simulink model "MicroGrid"  (R2021a)
settings: Solver=VariableStepAuto  StartTime=0  StopTime=24*3600  RelTol=1e-3
values from neighbouring files (symbols this model uses):
  A = A_prWindturbine * number_of_windturbines    (= 1530247.6)    [load_global_variables.m]
  Area_panels = 5*number_households    (= 1000000)    [load_global_variables.m]
  Battery_Capacity = 100e3    (= 100000)    [load_global_variables.m]
  controller_delay = 5    [load_global_variables.m]
  Efficiency_solar = 0.1    [load_global_variables.m]
  Efficiency_wind = 0.4    [load_global_variables.m]
  fuel_cell_power_rating = 50e6*4    (= 200000000)    [load_global_variables.m]
  H2_safety_buffer = 50e6    (= 50000000)    [load_global_variables.m]
  H2_selfsupply = 100e6    (= 100000000)    [load_global_variables.m]
  Max_H2_P_Input = 260000000    [load_global_variables.m]
  maxSOC = 100    [load_global_variables.m]
  Min_H2_P_Input = 1400    [load_global_variables.m]
  minSOC = 60    [load_global_variables.m]
  number_cars = number_households/3    (= 66666.6666667)    [load_global_variables.m]
  number_households = 200000    [load_global_variables.m]
  number_of_windturbines = 35    [load_global_variables.m]
  P_charge_max = 250e3    (= 250000)    [load_global_variables.m]
  P_rating_bat_single = 14e3    (= 14000)    [load_global_variables.m]
  Rho = 1.204    [load_global_variables.m]
  scenario = 5    [load_global_variables.m]
  SOC_safety_buffer = 80    [load_global_variables.m]
  SOC_selfsupply = 90    [load_global_variables.m]
  SOC_Start = 60    [load_global_variables.m]
  Start_Tank_Fill_L = 50e6    (= 50000000)    [load_global_variables.m]
  SunWinter = [0 0 0 0 0 0 0 33.54 130.49 211.47 234.96 271.04 ... (24 elements, 1x24)]    [SunWinter.mat]
undefined symbols (not defined in the file or in its folder): EV_dist, price, SunFall, SunSpring, SunSummer, Vind15nov, Vind23sep, wind
settings Model: Creator=cm  LastModifiedBy=cm

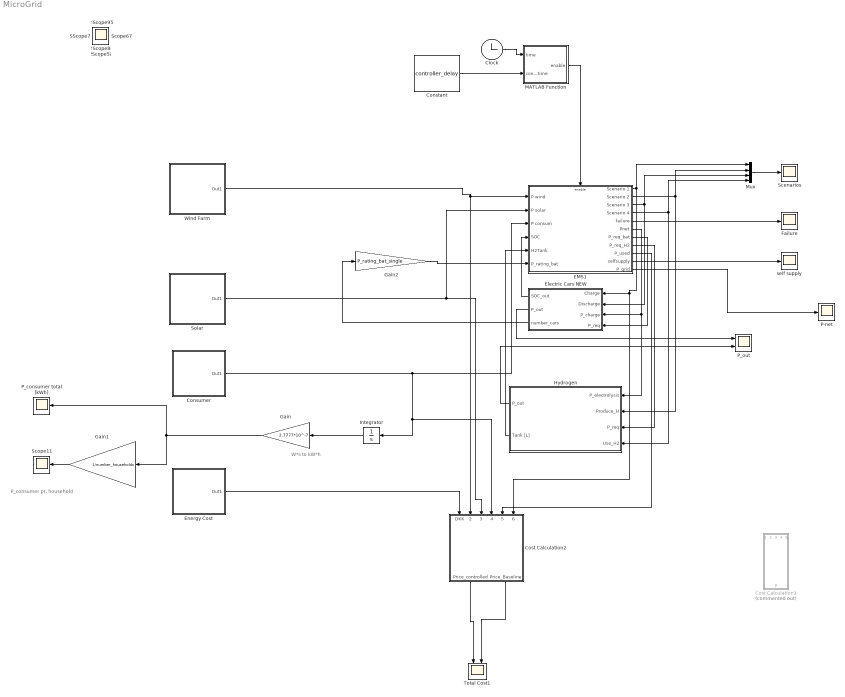
== system MicroGrid ==
  note: W*s to kW*h
  note: P_consumer pr. household
  Clock : Clock
  Constant : Constant  Value=controller_delay
  Consumer : Subsystem
      mask Display: image('C:\Users\cm\OneDrive - Danmarks Tekniske Universitet\Model-Based Systems Eng\05 Models\MBSE-MicroGrid\OurModel\Icons\House.png'); % Use "Edit Image" on toolstrip to change.
  Cost Calculation1 : Subsystem  Commented=on
  Cost Calculation2 : Subsystem
  EMS1 : Subsystem
  Electric Cars NEW : Subsystem
  Energy Cost : Subsystem
      mask Display: image('C:\Users\cm\OneDrive - Danmarks Tekniske Universitet\Model-Based Systems Eng\05 Models\MBSE-MicroGrid\OurModel\Icons\el_cost.png'); % Use "Edit Image" on toolstrip to change.
  Failure : Scope
  Gain : Gain  Gain=2.7777*10^-7
  Gain1 : Gain  Gain=1/number_households
  Gain2 : Gain  Gain=P_rating_bat_single
  Hydrogen : Subsystem
  Integrator : Integrator
  MATLAB Function : MATLAB Function  TreatAsAtomicUnit=on
  Mux : Mux
  P-net : Scope
  P_consumer total [kWh] : Scope
  P_out : Scope  NumInputPorts=2
  Scenarios : Scope
  Scope{,1..17} (18 alike) : Scope
  Solar : Subsystem
      mask Display: image('C:\Users\cm\OneDrive - Danmarks Tekniske Universitet\Model-Based Systems Eng\05 Models\MBSE-MicroGrid\OurModel\Icons\solar.png'); % Use "Edit Image" on toolstrip to change.
  Total Cost1 : Scope  NumInputPorts=2
  Wind Farm : Subsystem
      mask Display: image('C:\Users\cm\OneDrive - Danmarks Tekniske Universitet\Model-Based Systems Eng\05 Models\MBSE-MicroGrid\OurModel\Icons\wind.png'); % Use "Edit Image" on toolstrip to change.
  self supply : Scope
  wires:
  Electric Cars NEW/2(P_out) -> P_out/1
  Solar/1(Out1) -> Cost Calculation2/3(P solar), EMS1/2(P solar)
  EMS1/6(Pnet) -> Hydrogen/1(P_electrolysis), Electric Cars NEW/3(P_charge)
  EMS1/3(Scenario 3) -> Mux/3, Electric Cars NEW/2(Discharge)
  Hydrogen/2(Tank [L]) -> EMS1/5(H2Tank)
  Hydrogen/1(P_out) -> P_out/2
  Wind Farm/1(Out1) -> Cost Calculation2/2(P wind), EMS1/1(P wind)
  Electric Cars NEW/1(SOC_out) -> EMS1/4(SOC)
  Gain1/1 -> Scope11/1
  Gain/1 -> Gain1/1, P_consumer total [kWh]/1
  Energy Cost/1(Out1) -> Cost Calculation2/1(DKK)
  Integrator/1 -> Gain/1
  Cost Calculation2/1(Price_controlled) -> Total Cost1/1
  Consumer/1(Out1) -> EMS1/3(P consum), Cost Calculation2/4(P_consumer), Integrator/1
  Gain2/1 -> EMS1/6(P_rating_bat)
  Electric Cars NEW/3(number_cars) -> Gain2/1
  MATLAB Function/1(enable) -> EMS1/Enable
  Constant/1 -> MATLAB Function/2(controller_time)
  Clock/1 -> MATLAB Function/1(time)
  EMS1/1(Scenario 1) -> Mux/1, Cost Calculation2/6(P_cars), Electric Cars NEW/1(Charge)
  EMS1/2(Scenario 2) -> Mux/2, Hydrogen/2(Produce_H)
  EMS1/4(Scenario 4) -> Mux/4, Hydrogen/4(Use_H2)
  EMS1/5(failure) -> Failure/1
  EMS1/7(P_req_bat) -> Electric Cars NEW/4(P_req)
  EMS1/8(P_req_H2) -> Hydrogen/3(P_req)
  EMS1/10(selfsupply) -> self supply/1
  Cost Calculation2/2(Price_Baseline) -> Total Cost1/2
  EMS1/9(P_used) -> Cost Calculation2/5(P_used)
  EMS1/11(P_grid) -> P-net/1
  Mux/1 -> Scenarios/1

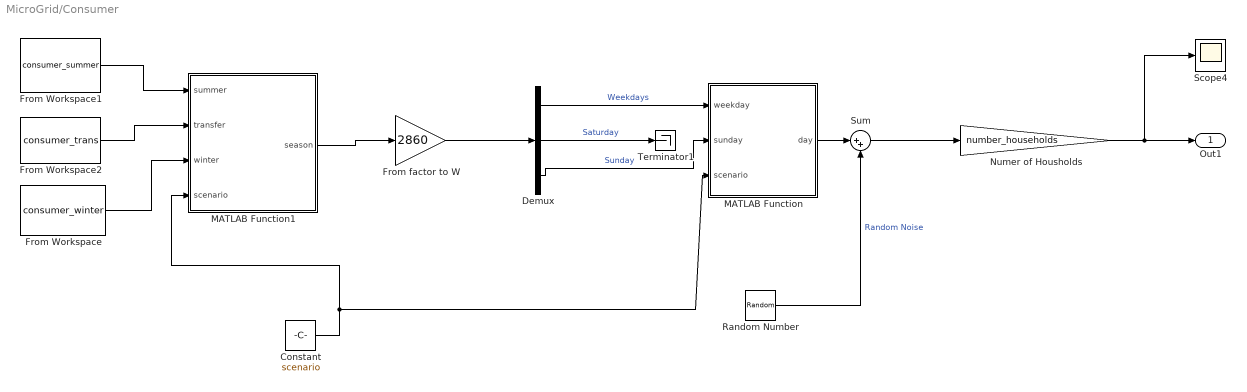
== system MicroGrid/Consumer ==
  Constant : Constant  Value=scenario
  Demux : Demux  Outputs=3
  From Workspace : FromWorkspace  VariableName=consumer_winter  SampleTime=24*60*60/96  Interpolate=off  ZeroCross=off  OutputAfterFinalValue=Cyclic repetition
  From Workspace1 : FromWorkspace  VariableName=consumer_summer  SampleTime=24*60*60/96  Interpolate=off  ZeroCross=off  OutputAfterFinalValue=Cyclic repetition
  From Workspace2 : FromWorkspace  VariableName=consumer_trans  SampleTime=24*60*60/96  Interpolate=off  ZeroCross=off  OutputAfterFinalValue=Cyclic repetition
  From factor to W : Gain  Gain=2860
  MATLAB Function : MATLAB Function  TreatAsAtomicUnit=on
  MATLAB Function1 : MATLAB Function  TreatAsAtomicUnit=on
  Numer of Housholds : Gain  Gain=number_households
  Random Number : RandomNumber  Variance=0.0001  SampleTime=1*60*60
  Scope4 : Scope
  Sum : Sum  Inputs=|++
  Terminator1 : Terminator
  Out1 : Outport
  wires:
  Demux/2 -> Terminator1/1  "Saturday"
  Random Number/1 -> Sum/2  "Random Noise"
  Demux/3 -> MATLAB Function/2(sunday)  "Sunday"
  Sum/1 -> Numer of Housholds/1
  Numer of Housholds/1 -> Out1/1, Scope4/1
  From factor to W/1 -> Demux/1
  From Workspace1/1 -> MATLAB Function1/1(summer)
  From Workspace2/1 -> MATLAB Function1/2(transfer)
  From Workspace/1 -> MATLAB Function1/3(winter)
  MATLAB Function1/1(season) -> From factor to W/1
  MATLAB Function/1(day) -> Sum/1
  Demux/1 -> MATLAB Function/1(weekday)  "Weekdays"
  Constant/1 -> MATLAB Function/3(scenario), MATLAB Function1/4(scenario)

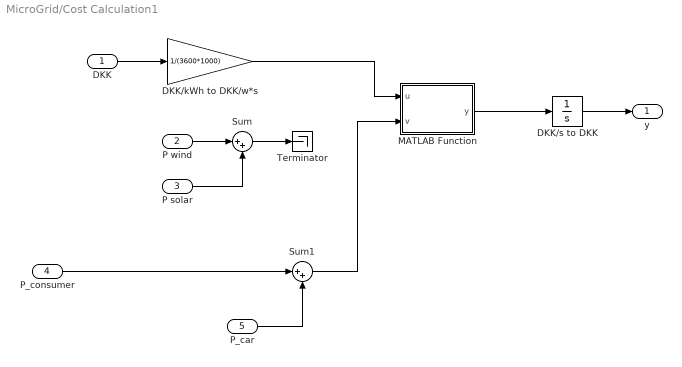
== system MicroGrid/Cost Calculation1 ==
  DKK : Inport
  P wind : Inport  Port=2
  P solar : Inport  Port=3
  P_consumer : Inport  Port=4
  P_car : Inport  Port=5
  DKK/kWh to DKK/w*s : Gain  Gain=1/(3600*1000)
  DKK/s to DKK : Integrator
  MATLAB Function : MATLAB Function  TreatAsAtomicUnit=on
  Sum : Sum  Inputs=|++
  Sum1 : Sum  Inputs=|++
  Terminator : Terminator
  y : Outport
  wires:
  P wind/1 -> Sum/1
  P solar/1 -> Sum/2
  MATLAB Function/1(y) -> DKK/s to DKK/1
  DKK/kWh to DKK/w*s/1 -> MATLAB Function/1(u)
  DKK/1 -> DKK/kWh to DKK/w*s/1
  DKK/s to DKK/1 -> y/1
  Sum/1 -> Terminator/1
  P_consumer/1 -> Sum1/1
  Sum1/1 -> MATLAB Function/2(v)
  P_car/1 -> Sum1/2

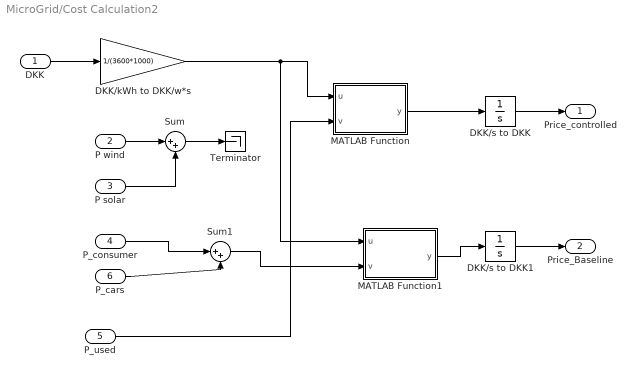
== system MicroGrid/Cost Calculation2 ==
  DKK : Inport
  P wind : Inport  Port=2
  P solar : Inport  Port=3
  P_consumer : Inport  Port=4
  P_used : Inport  Port=5
  P_cars : Inport  Port=6
  DKK/kWh to DKK/w*s : Gain  Gain=1/(3600*1000)
  DKK/s to DKK : Integrator
  DKK/s to DKK1 : Integrator
  MATLAB Function : MATLAB Function  TreatAsAtomicUnit=on
  MATLAB Function1 : MATLAB Function  TreatAsAtomicUnit=on
  Sum : Sum  Inputs=|++
  Sum1 : Sum  Inputs=|++
  Terminator : Terminator
  Price_controlled : Outport
  Price_Baseline : Outport  Port=2
  wires:
  P wind/1 -> Sum/1
  P solar/1 -> Sum/2
  MATLAB Function/1(y) -> DKK/s to DKK/1
  DKK/kWh to DKK/w*s/1 -> MATLAB Function1/1(u), MATLAB Function/1(u)
  DKK/1 -> DKK/kWh to DKK/w*s/1
  DKK/s to DKK/1 -> Price_controlled/1
  Sum/1 -> Terminator/1
  P_used/1 -> MATLAB Function/2(v)
  MATLAB Function1/1(y) -> DKK/s to DKK1/1
  DKK/s to DKK1/1 -> Price_Baseline/1
  P_cars/1 -> Sum1/2
  P_consumer/1 -> Sum1/1
  Sum1/1 -> MATLAB Function1/2(v)

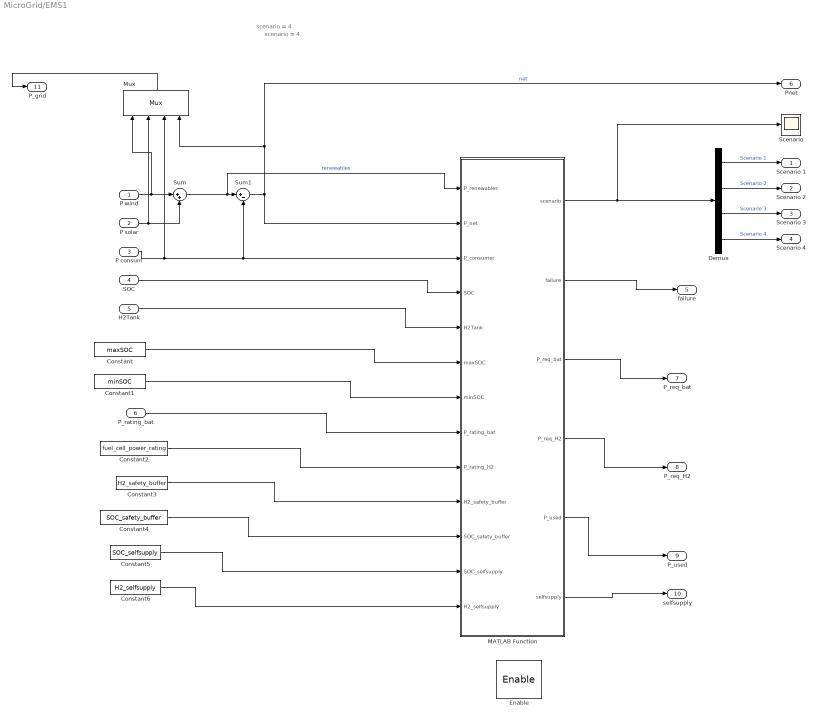
== system MicroGrid/EMS1 ==
  note: scenario = 4
  note: scenario = 4
  P wind : Inport
  P solar : Inport  Port=2
  P consum : Inport  Port=3
  SOC : Inport  Port=4
  H2Tank : Inport  Port=5
  P_rating_bat : Inport  Port=6
  Enable : EnablePort
  Constant : Constant  Value=maxSOC
  Constant1 : Constant  Value=minSOC
  Constant2 : Constant  Value=fuel_cell_power_rating
  Constant3 : Constant  Value=H2_safety_buffer
  Constant4 : Constant  Value=SOC_safety_buffer
  Constant5 : Constant  Value=SOC_selfsupply
  Constant6 : Constant  Value=H2_selfsupply
  Demux : Demux
  MATLAB Function : MATLAB Function  TreatAsAtomicUnit=on
  Mux : Mux
  Scenario : Scope
  Sum : Sum  Inputs=|++
  Sum1 : Sum  Inputs=|+-
  Scenario 1 : Outport
  Scenario 2 : Outport  Port=2
  Scenario 3 : Outport  Port=3
  Scenario 4 : Outport  Port=4
  failure : Outport  Port=5
  Pnet : Outport  Port=6
  P_req_bat : Outport  Port=7
  P_req_H2 : Outport  Port=8
  P_used : Outport  Port=9
  selfsupply : Outport  Port=10
  P_grid : Outport  Port=11
  wires:
  SOC/1 -> MATLAB Function/4(SOC)
  MATLAB Function/1(scenario) -> Scenario/1, Demux/1
  Demux/1 -> Scenario 1/1  "Scenario 1"
  Demux/2 -> Scenario 2/1  "Scenario 2"
  Demux/3 -> Scenario 3/1  "Scenario 3"
  Demux/4 -> Scenario 4/1  "Scenario 4"
  H2Tank/1 -> MATLAB Function/5(H2Tank)
  MATLAB Function/2(failure) -> failure/1
  Constant/1 -> MATLAB Function/6(maxSOC)
  Constant1/1 -> MATLAB Function/7(minSOC)
  MATLAB Function/3(P_req_bat) -> P_req_bat/1
  MATLAB Function/4(P_req_H2) -> P_req_H2/1
  Constant2/1 -> MATLAB Function/9(P_rating_H2)
  P_rating_bat/1 -> MATLAB Function/8(P_rating_bat)
  MATLAB Function/5(P_used) -> P_used/1
  Constant3/1 -> MATLAB Function/10(H2_safety_buffer)
  Constant4/1 -> MATLAB Function/11(SOC_safety_buffer)
  Constant5/1 -> MATLAB Function/12(SOC_selfsupply)
  Constant6/1 -> MATLAB Function/13(H2_selfsupply)
  P wind/1 -> Mux/1, Sum/1
  P solar/1 -> Sum/2, Mux/2
  Sum/1 -> MATLAB Function/1(P_renewables), Sum1/1  "renewables"
  P consum/1 -> Mux/3, Sum1/2, MATLAB Function/3(P_consumer)
  Sum1/1 -> MATLAB Function/2(P_net), Mux/4, Pnet/1  "net"
  MATLAB Function/6(selfsupply) -> selfsupply/1
  Mux/1 -> P_grid/1

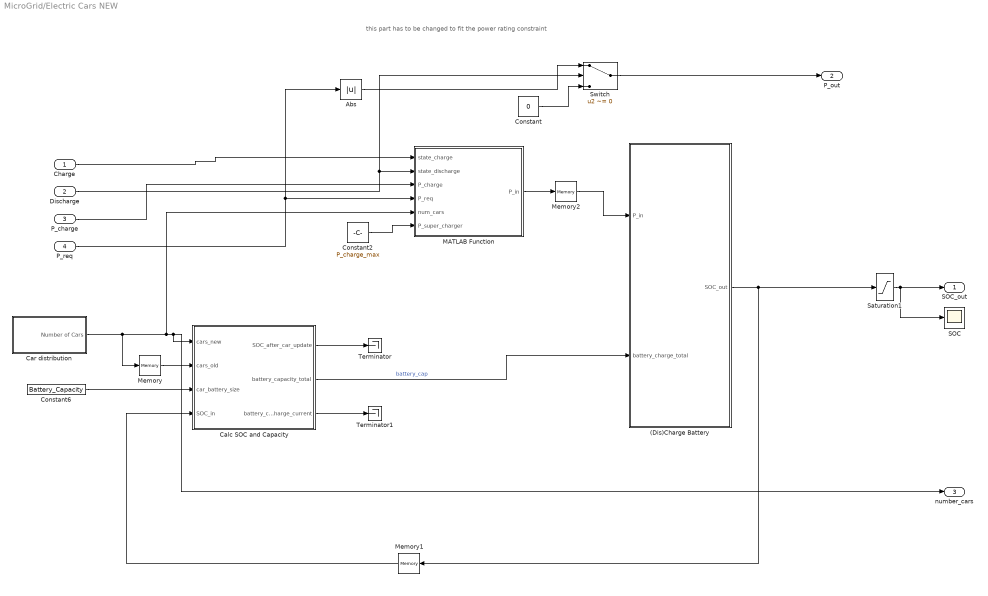
== system MicroGrid/Electric Cars NEW ==
  note: this part has to be changed to fit the power rating constraint
  Charge : Inport
  Discharge : Inport  Port=2
  P_charge : Inport  Port=3
  P_req : Inport  Port=4
  (Dis)Charge Battery : Subsystem
  Abs : Abs
  Calc SOC and Capacity : MATLAB Function  TreatAsAtomicUnit=on
  Car distribution : Subsystem  TreatAsAtomicUnit=on
  Constant : Constant  Value=0
  Constant2 : Constant  Value=P_charge_max
  Constant6 : Constant  Value=Battery_Capacity
  MATLAB Function : MATLAB Function  TreatAsAtomicUnit=on
  Memory : Memory  InitialCondition=EV_dist.signals.values(1) * number_cars
  Memory1 : Memory  InitialCondition=SOC_Start
  Memory2 : Memory
  SOC : Scope
  Saturation1 : Saturate  UpperLimit=100  LowerLimit=0
  Switch : Switch  Criteria=u2 ~= 0
  Terminator : Terminator
  Terminator1 : Terminator
  SOC_out : Outport
  P_out : Outport  Port=2
  number_cars : Outport  Port=3
  wires:
  Car distribution/1(Number of Cars) -> Memory/1, number_cars/1, Calc SOC and Capacity/1(cars_new), MATLAB Function/5(num_cars)
  Memory/1 -> Calc SOC and Capacity/2(cars_old)
  Constant6/1 -> Calc SOC and Capacity/3(car_battery_size)
  Memory1/1 -> Calc SOC and Capacity/4(SOC_in)
  MATLAB Function/1(P_in) -> Memory2/1
  Calc SOC and Capacity/2(battery_capacity_total) -> (Dis)Charge Battery/2(battery_charge_total)  "battery_cap"
  P_charge/1 -> MATLAB Function/3(P_charge)
  Discharge/1 -> Switch/2, MATLAB Function/2(state_discharge)
  Charge/1 -> MATLAB Function/1(state_charge)
  (Dis)Charge Battery/1(SOC_out) -> Saturation1/1, Memory1/1
  Abs/1 -> Switch/1
  Constant/1 -> Switch/3
  Memory2/1 -> (Dis)Charge Battery/1(P_in)
  Switch/1 -> P_out/1
  P_req/1 -> Abs/1, MATLAB Function/4(P_req)
  Saturation1/1 -> SOC_out/1, SOC/1
  Constant2/1 -> MATLAB Function/6(P_super_charger)
  Calc SOC and Capacity/1(SOC_after_car_update) -> Terminator/1
  Calc SOC and Capacity/3(battery_charge_current) -> Terminator1/1

== system MicroGrid/Energy Cost ==
  From Workspace : FromWorkspace  VariableName=price  SampleTime=24*60*60/length(price.signals.values)  Interpolate=off  ZeroCross=off  OutputAfterFinalValue=Cyclic repetition
  Out1 : Outport
  wires:
  From Workspace/1 -> Out1/1

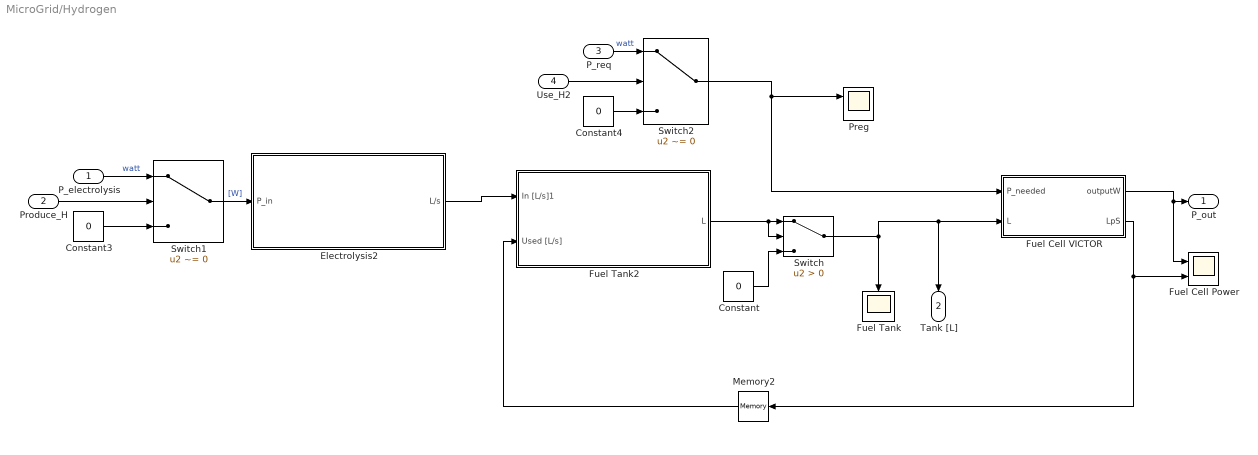
== system MicroGrid/Hydrogen ==
  P_electrolysis : Inport
  Produce_H : Inport  Port=2
  P_req : Inport  Port=3
  Use_H2 : Inport  Port=4
  Constant : Constant  Value=0
  Constant3 : Constant  Value=0
  Constant4 : Constant  Value=0
  Electrolysis2 : Subsystem
  Fuel Cell Power : Scope  NumInputPorts=2
  Fuel Cell VICTOR : Subsystem
  Fuel Tank : Scope
  Fuel Tank2 : Subsystem
  Memory2 : Memory
  Preg : Scope  NumInputPorts=2
  Switch : Switch  Criteria=u2 > Threshold
  Switch1 : Switch  Criteria=u2 ~= 0  Threshold=1
  Switch2 : Switch  Criteria=u2 ~= 0  Threshold=1
  P_out : Outport
  Tank [L] : Outport  Port=2
  wires:
  Fuel Tank2/1(L) -> Switch/2, Switch/1
  Memory2/1 -> Fuel Tank2/2(Used [L/s])
  Electrolysis2/1(L/s) -> Fuel Tank2/1(In [L/s]1)
  Fuel Cell VICTOR/2(LpS) -> Fuel Cell Power/2, Memory2/1
  Constant3/1 -> Switch1/3
  P_electrolysis/1 -> Switch1/1  "watt"
  Switch1/1 -> Electrolysis2/1(P_in)  "[W]"
  Produce_H/1 -> Switch1/2
  P_req/1 -> Switch2/1  "watt"
  Use_H2/1 -> Switch2/2
  Constant4/1 -> Switch2/3
  Switch2/1 -> Preg/1, Fuel Cell VICTOR/1(P_needed)
  Fuel Cell VICTOR/1(outputW) -> Fuel Cell Power/1, P_out/1
  Switch/1 -> Tank [L]/1, Fuel Cell VICTOR/2(L), Fuel Tank/1
  Constant/1 -> Switch/3

== system MicroGrid/Solar ==
  note: Efficiency: 10%
      | Area: 80.000 m2
      | No shadow
  Irradiance : Subsystem
      mask init:
      | load power_V2G
      mask Display: plot(V2G.IRRADIANCE.time,V2G.IRRADIANCE.SUN)
  Power [W] : Scope
  Rate Limiter2 : RateLimiter  RisingSlewLimit=1e4  FallingSlewLimit=-1e4  SampleTimeMode=inherited
  efficiency : Gain  Gain=Efficiency_solar
  m2 : Gain  Gain=Area_panels
  Out1 : Outport
  wires:
  Irradiance/1(" ") -> Rate Limiter2/1
  m2/1 -> efficiency/1
  efficiency/1 -> Out1/1, Power [W]/1
  Rate Limiter2/1 -> m2/1

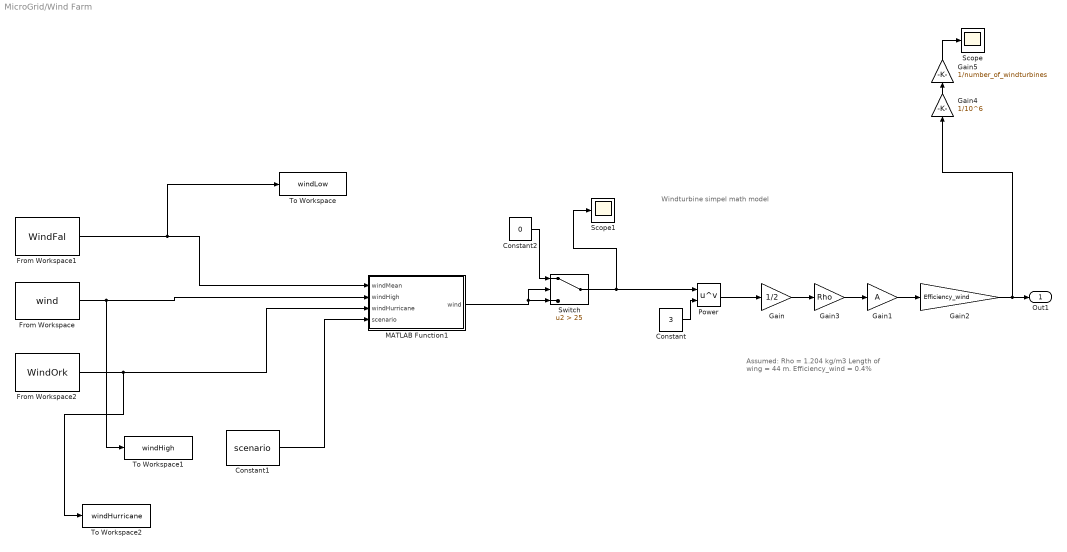
== system MicroGrid/Wind Farm ==
  note: Assumed:
      | Rho = 1.204 kg/m3
      | Length of wing = 44 m.
      | Efficiency_wind = 0.4%
  note: Windturbine simpel math model
  Constant : Constant  Value=3
  Constant1 : Constant  Value=scenario
  Constant2 : Constant  Value=0
  From Workspace : FromWorkspace  VariableName=wind  SampleTime=24*60*60/(length(wind.signals.values))  Interpolate=off  ZeroCross=off  OutputAfterFinalValue=Cyclic repetition
  From Workspace1 : FromWorkspace  VariableName=WindFal  SampleTime=24*60*60/(length(Vind15nov))  Interpolate=off  ZeroCross=off  OutputAfterFinalValue=Cyclic repetition
  From Workspace2 : FromWorkspace  VariableName=WindOrk  SampleTime=24*60*60/(length(Vind23sep))  Interpolate=off  ZeroCross=off  OutputAfterFinalValue=Cyclic repetition
  Gain : Gain  Gain=1/2
  Gain1 : Gain  Gain=A
  Gain2 : Gain  Gain=Efficiency_wind
  Gain3 : Gain  Gain=Rho
  Gain4 : Gain  Gain=1/10^6
  Gain5 : Gain  Gain=1/number_of_windturbines
  MATLAB Function1 : MATLAB Function  TreatAsAtomicUnit=on
  Power : Math  Operator=pow  SaturateOnIntegerOverflow=on
  Scope : Scope
  Scope1 : Scope
  Switch : Switch  Criteria=u2 > Threshold  Threshold=25
  To Workspace : ToWorkspace  VariableName=windLow  SaveFormat=Timeseries  SampleTime=-1
  To Workspace1 : ToWorkspace  VariableName=windHigh  SaveFormat=Timeseries  SampleTime=-1
  To Workspace2 : ToWorkspace  VariableName=windHurricane  SaveFormat=Timeseries  SampleTime=-1
  Out1 : Outport
  wires:
  Power/1 -> Gain/1
  Gain1/1 -> Gain2/1
  Constant/1 -> Power/2
  Gain/1 -> Gain3/1
  Gain3/1 -> Gain1/1
  Gain2/1 -> Gain4/1, Out1/1
  Switch/1 -> Scope1/1, Power/1
  Constant2/1 -> Switch/1
  MATLAB Function1/1(wind) -> Switch/2, Switch/3
  From Workspace1/1 -> To Workspace/1, MATLAB Function1/1(windMean)
  From Workspace/1 -> MATLAB Function1/2(windHigh), To Workspace1/1
  From Workspace2/1 -> To Workspace2/1, MATLAB Function1/3(windHurricane)
  Constant1/1 -> MATLAB Function1/4(scenario)
  Gain5/1 -> Scope/1
  Gain4/1 -> Gain5/1

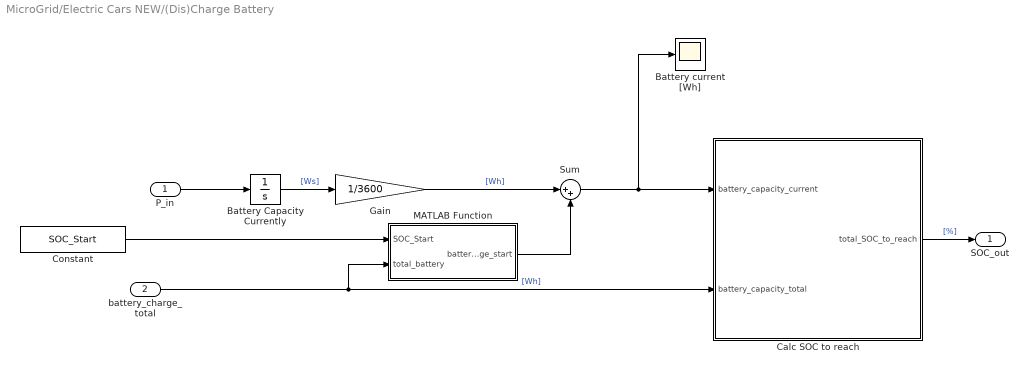
== system MicroGrid/Electric Cars NEW/(Dis)Charge Battery ==
  P_in : Inport
  battery_charge_total : Inport  Port=2
  Battery Capacity Currently : Integrator
  Battery current [Wh] : Scope
  Calc SOC to reach : MATLAB Function  TreatAsAtomicUnit=on
  Constant : Constant  Value=SOC_Start
  Gain : Gain  Gain=1/3600
  MATLAB Function : MATLAB Function  TreatAsAtomicUnit=on
  Sum : Sum  Inputs=|++
  SOC_out : Outport
  wires:
  battery_charge_total/1 -> Calc SOC to reach/2(battery_capacity_total), MATLAB Function/2(total_battery)  "[Wh]"
  Calc SOC to reach/1(total_SOC_to_reach) -> SOC_out/1  "[%]"
  Battery Capacity Currently/1 -> Gain/1  "[Ws]"
  Gain/1 -> Sum/1  "[Wh]"
  Sum/1 -> Battery current [Wh]/1, Calc SOC to reach/1(battery_capacity_current)
  MATLAB Function/1(battery_charge_start) -> Sum/2
  P_in/1 -> Battery Capacity Currently/1
  Constant/1 -> MATLAB Function/1(SOC_Start)

== system MicroGrid/Electric Cars NEW/Car distribution ==
  From Workspace : FromWorkspace  VariableName=EV_dist  SampleTime=24*60*60/length(EV_dist.signals.values)  Interpolate=off  ZeroCross=off  OutputAfterFinalValue=Cyclic repetition
  Gain : Gain  Gain=number_cars
  Number of cars : Scope
  Round : Rounding  Operator=round
  Number of Cars : Outport
  wires:
  Round/1 -> Number of Cars/1, Number of cars/1
  Gain/1 -> Round/1
  From Workspace/1 -> Gain/1  "[%]"

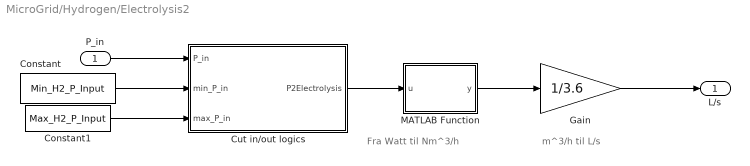
== system MicroGrid/Hydrogen/Electrolysis2 ==
  note: m^3/h til L/s
  note: Fra Watt til Nm^3/h
  P_in : Inport
  Constant : Constant  Value=Min_H2_P_Input
  Constant1 : Constant  Value=Max_H2_P_Input
  Cut in/out logics : MATLAB Function  TreatAsAtomicUnit=on
  Gain : Gain  Gain=1/3.6
  MATLAB Function : MATLAB Function  TreatAsAtomicUnit=on
  L/s : Outport
  wires:
  P_in/1 -> Cut in/out logics/1(P_in)
  Constant/1 -> Cut in/out logics/2(min_P_in)
  Constant1/1 -> Cut in/out logics/3(max_P_in)
  Cut in/out logics/1(P2Electrolysis) -> MATLAB Function/1(u)
  MATLAB Function/1(y) -> Gain/1
  Gain/1 -> L/s/1

== system MicroGrid/Hydrogen/Fuel Cell VICTOR ==
  note: [W]
  P_needed : Inport
  L : Inport  Port=2
  Constant4 : Constant  Value=fuel_cell_power_rating
  MATLAB Function3 : MATLAB Function  TreatAsAtomicUnit=on
  outputW : Outport
  LpS : Outport  Port=2
  wires:
  MATLAB Function3/1(P_out) -> outputW/1
  L/1 -> MATLAB Function3/3(Liter)
  MATLAB Function3/2(LpS_out) -> LpS/1
  P_needed/1 -> MATLAB Function3/1(P_needed)
  Constant4/1 -> MATLAB Function3/2(fuel_cell_power_rating)

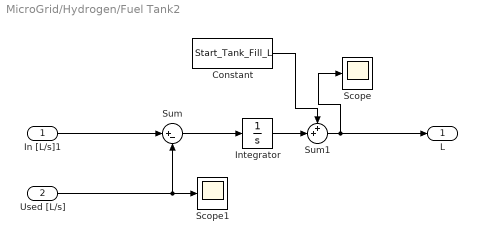
== system MicroGrid/Hydrogen/Fuel Tank2 ==
  In [L/s]1 : Inport
  Used [L/s] : Inport  Port=2
  Constant : Constant  Value=Start_Tank_Fill_L
  Integrator : Integrator
  Scope : Scope
  Scope1 : Scope
  Sum : Sum  Inputs=|+-
  Sum1 : Sum  Inputs=++|
  L : Outport
  wires:
  Used [L/s]/1 -> Scope1/1, Sum/2
  In [L/s]1/1 -> Sum/1
  Sum/1 -> Integrator/1
  Integrator/1 -> Sum1/2
  Sum1/1 -> Scope/1, L/1
  Constant/1 -> Sum1/1

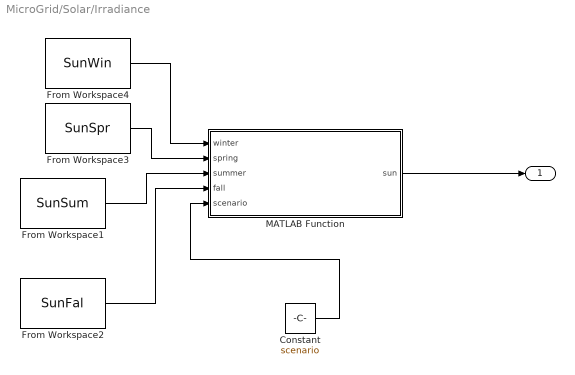
== system MicroGrid/Solar/Irradiance ==
  Constant : Constant  Value=scenario
  From Workspace1 : FromWorkspace  VariableName=SunSum  SampleTime=24*60*60/(length(SunSummer))  Interpolate=off  ZeroCross=off  OutputAfterFinalValue=Cyclic repetition
  From Workspace2 : FromWorkspace  VariableName=SunFal  SampleTime=24*60*60/(length(SunFall))  Interpolate=off  ZeroCross=off  OutputAfterFinalValue=Cyclic repetition
  From Workspace3 : FromWorkspace  VariableName=SunSpr  SampleTime=24*60*60/(length(SunSpring))  Interpolate=off  ZeroCross=off  OutputAfterFinalValue=Cyclic repetition
  From Workspace4 : FromWorkspace  VariableName=SunWin  SampleTime=24*60*60/(length(SunWinter))  Interpolate=off  ZeroCross=off  OutputAfterFinalValue=Cyclic repetition
  MATLAB Function : MATLAB Function  TreatAsAtomicUnit=on
  " " : Outport  VectorParamsAs1DForOutWhenUnconnected=off
  wires:
  From Workspace1/1 -> MATLAB Function/3(summer)
  From Workspace2/1 -> MATLAB Function/4(fall)
  From Workspace3/1 -> MATLAB Function/2(spring)
  From Workspace4/1 -> MATLAB Function/1(winter)
  MATLAB Function/1(sun) -> " "/1
  Constant/1 -> MATLAB Function/5(scenario)

== matlab function MicroGrid/Cost Calculation2/MATLAB Function ==
  data: u input; y output; v input
function y = multiply(u,v)

y = u*v;

== matlab function MicroGrid/Cost Calculation2/MATLAB Function1 ==
  data: u input; y output; v input
function y = multiply(u,v)

y = u*v;

== matlab function MicroGrid/Wind Farm/MATLAB Function1 ==
  data: windMean input; wind output; windHigh input; windHurricane input; scenario input
function wind = fcn(windMean, windHigh, windHurricane, scenario)


if scenario == 1
    wind = windMean;


elseif scenario == 2
    wind = windHurricane;


elseif scenario == 3
    wind = windMean;


elseif scenario == 4
    wind = windHigh;


elseif scenario == 5
    wind = windMean;


elseif scenario == 6
    wind = windMean;
    
else
    wind = windMean;

end

== matlab function MicroGrid/Electric Cars NEW/MATLAB Function ==
  data: state_charge input; P_in output; state_discharge input; P_charge input; P_req input; num_cars input; P_super_charger input
function P_in = fcn(state_charge, state_discharge, P_charge, P_req, num_cars, P_super_charger)

% function takes care that P_in is negative if we discharge and positive if
% we charge

if state_charge == 1
    P_in = abs(P_charge);
    P_possible = num_cars * P_super_charger;
    if P_in > P_possible
        P_in = P_possible;
        disp('Battery: P_in_limit reached')
    end
elseif state_discharge == 1
    P_in = -abs(P_req);
else
    P_in = 0;
end

== matlab function MicroGrid/Electric Cars NEW/(Dis)Charge Battery/MATLAB Function ==
  data: SOC_Start input; battery_charge_start output; total_battery input
function battery_charge_start = fcn(SOC_Start, total_battery)

battery_charge_start = SOC_Start/100 * total_battery;

== matlab function MicroGrid/Consumer/MATLAB Function1 ==
  data: summer input; season output; transfer input; winter input; scenario input
function season = fcn(summer, transfer, winter, scenario)


if scenario == 1
    season = summer;

elseif scenario == 2
    season = transfer;

elseif scenario == 3
    season = winter;


elseif scenario == 4
    season = winter;

elseif scenario == 5
    season = transfer;

elseif scenario == 6
    season = winter;
    
else
    season = summer;
end

== matlab function MicroGrid/Hydrogen/Electrolysis2/Cut in//out logics ==
  data: P_in input; min_P_in input; P2Electrolysis output; max_P_in input
function P2Electrolysis = fcn(P_in, min_P_in, max_P_in)

if P_in >= min_P_in && P_in <= max_P_in
    
    P2Electrolysis = P_in;
elseif P_in > max_P_in
    P2Electrolysis = max_P_in;
elseif P_in < min_P_in
    P2Electrolysis = 0;
else
    % case shouldnt happen, but to secure our butts
    P2Electrolysis = max_P_in;
end

== matlab function MicroGrid/Hydrogen/Electrolysis2/MATLAB Function ==
  data: u input; y output
function y = fcn(u)
 
%Værdier for min og maks Elektrolyse 
% https://cellar-c2.services.clever-cloud.com/com-mcphy/uploads/2020/08/20.05.McPhy_Portfolio_ELY_Piel_EN.pdf
%x2=2
%x1=1

%y2=4.4*10
%y1=2.4


%a=(log(y2)-log(y1))/(log(x2)-log(x1))

%b=y1/(x1^a)
%y=b*u^a

x1=0;
x2=570000;  %[W]

y1=0;
y2=150; %[m3/h]

a=(y2-y1)/(x2-x1);
b=y1-a*x1;


y=a*u+b;

== matlab function MicroGrid/Hydrogen/Fuel Cell VICTOR/MATLAB Function3 ==
  data: P_needed input; fuel_cell_power_rating input; Liter input; P_out output; LpS_out output
function [P_out,LpS_out]  = fcn(P_needed, fuel_cell_power_rating, Liter)

P_needed = abs(P_needed);
%Her omdaner vi fra H2 L til W
x1=0;
x2=0.22333333333;

y1=0;
y2=1000;

a=(y2-y1)/(x2-x1);
b=y1-a*x1;

%Dette er så meget hydrogen vi max kan bruge!
max_P_out_Ls =  (fuel_cell_power_rating-b)/ a;

%Dette er så meget hydrogen vi skal bruge lige nu!
Ls_needed=(P_needed-b)/a;


if fuel_cell_power_rating > P_needed && Liter > Ls_needed   
    P_out = P_needed;
    LpS_out = (P_needed-b)/a;
    LpS_out = abs(LpS_out); 
    
elseif fuel_cell_power_rating < P_needed && Liter > Ls_needed
    P_out = fuel_cell_power_rating;
    LpS_out = (fuel_cell_power_rating-b)/a;
    LpS_out = abs(LpS_out); 
    
elseif fuel_cell_power_rating > P_needed && Liter < Ls_needed
    P_out = a*Liter+b;
    LpS_out = (Liter-b)/a;
    LpS_out = abs(LpS_out); 
    
else
    P_out = 0;
    LpS_out =0;

end


%Her vil den give et output hele tiden! Hvilket er dårligt!
%LpS_out = (P_needed-b)/ a;  


end

== matlab function MicroGrid/Solar/Irradiance/MATLAB Function ==
  data: winter input; sun output; spring input; summer input; fall input; scenario input
function sun = fcn(winter, spring, summer, fall, scenario)

if scenario == 1
    sun = summer;


elseif scenario == 2
    sun = fall;


elseif scenario == 3
    sun = winter;


elseif scenario == 4
    sun = summer;


elseif scenario == 5
    sun = spring;


elseif scenario == 6
    sun = winter;
    
else
    sun = summer;

end

== matlab function MicroGrid/Cost Calculation1/MATLAB Function ==
  data: u input; y output; v input
function y = multiply(u,v)

y = u*v;

== matlab function MicroGrid/EMS1/MATLAB Function ==
  data: P_renewables input; P_net input; P_consumer input; scenario output; SOC input; H2Tank input; failure output; maxSOC input; minSOC input; P_rating_bat input; P_rating_H2 input; P_req_bat output; P_req_H2 output; H2_safety_buffer input; SOC_safety_buffer input; P_used output; SOC_selfsupply input; H2_selfsupply input; selfsupply output
function [scenario,failure, P_req_bat, P_req_H2, P_used, selfsupply ] = fcn(P_renewables, P_net, P_consumer, SOC, H2Tank, maxSOC, minSOC,...
    P_rating_bat, P_rating_H2, H2_safety_buffer, SOC_safety_buffer, SOC_selfsupply, H2_selfsupply)

scenario = [0,0,0,0];
failure = 0;

% Self Supplying logic

% for godlike controller we can analyise the total price and make a smart
% decision on when to be self supplying. This part could be our
% optimisation.

if SOC > SOC_selfsupply && H2Tank > H2_selfsupply
    selfsupply = true;
else
    selfsupply = false;
end

% Heuristics
if selfsupply == true
    P_used = 0;
    % supply consumer with energy from system
    P_req_bat = abs(P_consumer);
    P_req_H2 = abs(P_consumer);
    % First use Hydrogen and afterwards use batteries
    % more energy consumed than produced
    
    if abs(P_consumer) <= P_rating_H2 + P_rating_bat
        % conumption can be covered only by using the stored energy
        
        % Use Hydrogen first
        if H2Tank > H2_safety_buffer
            scenario = [0 0 0 1];
            if abs(P_consumer) > P_rating_H2
                % also use battery
                scenario = [0 0 1 1];
                P_req_H2 = P_rating_H2;
                P_req_bat = abs(P_consumer) - P_rating_H2;
            end
            % Use Battery
        elseif SOC > SOC_safety_buffer
            scenario = [0 0 1 0];
            if abs(P_consumer) > P_rating_bat
                % also use Hydrogen
                scenario = [0 0 1 1];
                P_req_bat = P_rating_bat;
                P_req_H2 = abs(P_consumer) - P_rating_bat;
            end
        else
            error('selfsupply: Power rating problem. Case not implemented')
        end
        % P_consumer > P_rating -> use some of the net as well.
    elseif abs(P_consumer) > P_rating_H2 + P_rating_bat
        % P_consumer > P_rating -> use some of the net as well.
        P_req_bat = P_rating_bat;
        P_req_H2 = P_rating_H2;
        P_used = abs(P_consumer) - P_req_bat - P_req_H2;
        
    else
        error('selfsupply: Power rating case not implemented')
        
    end % Power rating
    
else
    % selfsupply == false
    P_used = P_renewables;
    
    if P_net == 0
        scenario = [0 0 0 0];
        P_req_bat = 0;
        P_req_H2 = 0;
        % more engery produced than consumed
    elseif P_net > 0
        P_req_bat = 0;
        P_req_H2 = 0;
        % Battery under min limit
        if SOC < SOC_safety_buffer
            scenario = [1 0 0 0]; % charge battery
        elseif H2Tank < H2_safety_buffer
            scenario = [0 1 0 0]; % Produce Hydrogen
            
        elseif H2Tank >= H2_safety_buffer && SOC < maxSOC
            scenario = [1 0 0 0]; % charge battery
            % Battery full
        elseif SOC >= maxSOC
            % Poduce Hydrogen
            scenario = [0 1 0 0];
        else
            error('Battery charge case missing')
        end % Battery charging
        
        % more energy consumed than produced
    elseif P_net < 0
        P_req_bat = abs(P_net);
        P_req_H2 = abs(P_net);
        % Check power rating
        if abs(P_net) > P_rating_bat + P_rating_H2
            scenario = [0 0 0 0];
            % required P bigger than what we can supply
            failure = 1;
            disp('Blackout: max P out limit reached')
            % Tank not at lower bound
        elseif H2Tank >= H2_safety_buffer
            % Use Hydrogen
            
            scenario = [0 0 0 1];
            P_req_bat = 0;
            P_req_H2 = abs(P_net);
            % cant supply all the power needed
            if P_rating_H2 > P_req_H2
                % do nothing. This is just to cover that we dont get the
                % error
            elseif P_rating_H2 <= P_req_H2 && SOC > 0
                scenario = [0 0 1 1];
                P_req_H2 = P_rating_H2;
                P_req_bat = abs(P_net)-P_req_H2;
            elseif P_rating_H2 <= P_req_H2 && SOC <= 0
                scenario = [0 0 0 0];
                failure = 1;
                disp('Blackout: P rating H2 reached and no Battery left')
            else
                error('Grid supply (H2 use): Case not implemented')
            end % power rating
            
        elseif H2Tank < H2_safety_buffer
            if SOC >= minSOC
                % Take the rest out of the battery
                scenario = [0 0 1 0];
                P_req_bat = abs(P_net);
                P_req_H2 = 0;
                
                if P_rating_bat <= P_req_bat && H2Tank > 0
                    % cant supply all the power needed
                    scenario = [0 0 1 1];
                    P_req_bat = P_rating_bat;
                    P_req_H2 = abs(P_net)-P_req_H2;
                elseif P_rating_bat <= P_req_bat && H2Tank <= 0
                    scenario = [0 0 0 0];
                    failure = 1;
                    disp('Blackout: P rating bat reached and no H2 left')
                end
                
                
            elseif SOC < minSOC && H2Tank > 0
                % use rest of Hydrogen
                scenario = [0 0 0 1];
                P_req_bat = 0;
                P_req_H2 = abs(P_net);
                
                % cant supply all the power needed
                if P_rating_H2 <= P_req_H2 && SOC > 0
                    scenario = [0 0 1 1];
                    P_req_H2 = P_rating_H2;
                    P_req_bat = abs(P_net)-P_req_H2;
                elseif P_rating_H2 <= P_req_H2 && SOC <= 0
                    scenario = [0 0 0 0];
                    failure = 1;
                    disp('Blackout: P rating H2 reached and no Battery left')
                end
                
                
            elseif SOC < minSOC && SOC > 0 && H2Tank <= 0
                % use the rest of the Battery
                scenario = [0 0 1 0];
                P_req_bat = abs(P_net);
                P_req_H2 = 0;
                if P_rating_bat <= P_req_bat
                    scenario = [0 0 0 0];
                    failure = 1;
                    disp('Blackout: Not enough P rating in Battery and H2 empty')
                end
            else
                error('Use Battery: case missing')
                
            end  % Battery
            
        end % Hydrogen
        
    else
        error('missing a case in EMS')
        
    end % Grid supply outer
end

% pause(controller_delay)
end

== matlab function MicroGrid/MATLAB Function ==
  data: time input; enable output; controller_time input
function enable = fcn(time,controller_time)

if mod(time,controller_time)== 0
    enable = 1;
else
    enable = 0;
end
end

== matlab function MicroGrid/Consumer/MATLAB Function ==
  data: weekday input; day output; sunday input; scenario input
function day = fcn(weekday, sunday, scenario)


if scenario == 1
    day = weekday;

elseif scenario == 2
    day = weekday;


elseif scenario == 3
    day = weekday;


elseif scenario == 4
    day = weekday;


elseif scenario == 5
    day = sunday;


elseif scenario == 6
    day = weekday;
    
else
    day = weekday;
end

== matlab function MicroGrid/Electric Cars NEW/(Dis)Charge Battery/Calc SOC to reach ==
  data: battery_capacity_current input; total_SOC_to_reach output; battery_capacity_total input
function total_SOC_to_reach = fcn(battery_capacity_current, battery_capacity_total)


total_SOC_to_reach = (battery_capacity_current / battery_capacity_total) * 100;

== matlab function MicroGrid/Electric Cars NEW/Calc SOC and Capacity ==
  data: cars_new input; SOC_after_car_update output; cars_old input; car_battery_size input; SOC_in input; battery_capacity_total output; battery_charge_current output
function [SOC_after_car_update, battery_capacity_total, battery_charge_current]  = fcn(cars_new, cars_old, car_battery_size, SOC_in)

% For now we we see the cars as one and just a distribution over all
% IDEA:
    % We could work with cars as an array, each car is an element of the array
    % is a car. If the car is not in the charger the specific element in the
    % array is 0 otherwise it indicates the SOC.
    % Then we need a Controller in the Electric car model which loads the cars
    % individually

if cars_old == cars_new
    SOC_after_car_update = SOC_in;
elseif cars_old < cars_new
    % more cars
    % Calculate SOC of new cars randomly
    std_dev = 15;
    mean = 35;
    SOC_new = std_dev.*randn(1) + mean;
    
    if SOC_new <= 0
        % might happen because of normal distribution
        SOC_new = 1;
    end
    
    % Calculate new battery charge
    num_new_cars = cars_new - cars_old;
    capacity_new_cars = SOC_new/100 * car_battery_size * num_new_cars;
    
    capacity_old_cars = SOC_in/100 * car_battery_size * cars_old;
    
    % Calc SOC = (cap_new + cap_old) / total_cap * 100%
    SOC_after_car_update = (capacity_old_cars+capacity_new_cars)/(car_battery_size*cars_new) * 100;
    
elseif cars_old > cars_new
    % less cars
    SOC_after_car_update = SOC_in; % dont know how to do it otherwise, ideas welcome
    

else 
    % should not happen
    error('In Electric Cars/SOCcalc: unexpected case')
    SOC_after_car_update = SOC_in;
end



battery_capacity_total = car_battery_size * cars_new;
battery_charge_current = SOC_after_car_update/100 * battery_capacity_total;
